simulink model "GSFR_Individual_Vars"  (R2019b)
settings: Solver=VariableStepAuto  StartTime=0  StopTime=20.0  MaxStep=0.01  RelTol=1e-3
model workspace (MAT data in the model file):
  H = [8 1]
values from neighbouring files (symbols this model uses):
  c = (((2*H*R)+(((D*R)+(K*Fh))*Tr))/(2*(D*R+K)))*wn    [Monte_Carlo_Half_Injection.m]    (also in Range_H_Half_Injection.m; Range_H_Ideal_Injection.m)
  D = 1.0    (= 1)    [Monte_Carlo_Half_Injection.m]    (also in Range_H_Half_Injection.m; Range_H_Ideal_Injection.m)
  Fh = 0.034*randn()+0.25    [Monte_Carlo_Half_Injection.m]    (also in Range_H_Half_Injection.m = 0.2; Range_H_Ideal_Injection.m = 0.4)
  K = 0.95    [Monte_Carlo_Half_Injection.m]    (also in Range_H_Half_Injection.m = 0.8; Range_H_Ideal_Injection.m = 1)
  Pd = -0.1    [Monte_Carlo_Half_Injection.m]    (also in Range_H_Half_Injection.m; Range_H_Ideal_Injection.m)
  R = (0.05/3)*randn()+0.075    [Monte_Carlo_Half_Injection.m]    (also in Range_H_Half_Injection.m = 0.075; Range_H_Ideal_Injection.m = 0.04)
  Tr = 0.67*randn()+9    [Monte_Carlo_Half_Injection.m]    (also in Range_H_Half_Injection.m = 8; Range_H_Ideal_Injection.m = 8)
  wn = sqrt((D*R+K)/(2*H*R*Tr))    [Monte_Carlo_Half_Injection.m]    (also in Range_H_Half_Injection.m; Range_H_Ideal_Injection.m)
settings Model: EnablePacing=on  PacingRate=1000  ParameterArgumentNames=H  OrderedModelArguments=off  Creator=ruiva  LastModifiedBy=ruiva

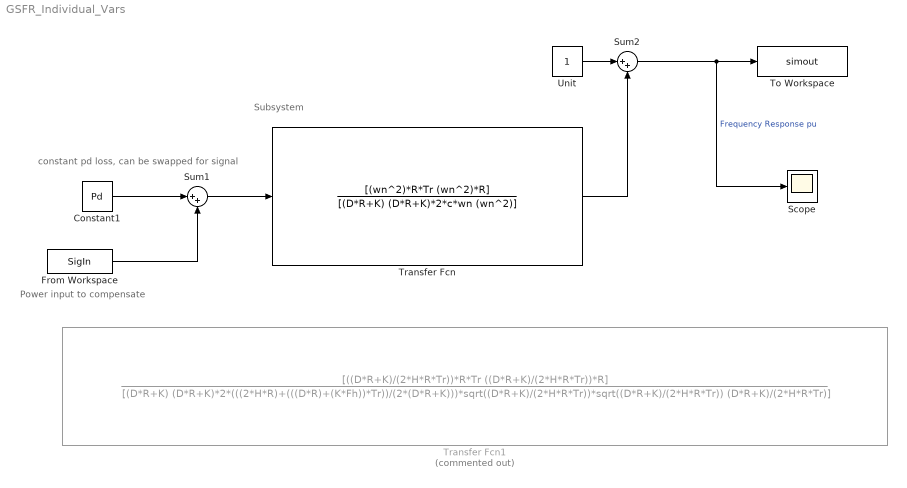
== system GSFR_Individual_Vars ==
  note: Subsystem
  note: Power input to compensate
  note: constant pd loss, can be swapped for signal
  Constant1 : Constant  Value=Pd
  From Workspace : FromWorkspace  VariableName=SigIn  SampleTime=0
  Scope : Scope
  Sum1 : Sum  Inputs=|++
  Sum2 : Sum  Inputs=|++
  To Workspace : ToWorkspace  VariableName=simout  SaveFormat=Timeseries  SampleTime=-1
  Transfer Fcn : TransferFcn  Numerator=[(wn^2)*R*Tr (wn^2)*R]  Denominator=[(D*R+K) (D*R+K)*2*c*wn (wn^2)]
  Transfer Fcn1 : TransferFcn  Commented=on  Numerator=[((D*R+K)/(2*H*R*Tr))*R*Tr ((D*R+K)/(2*H*R*Tr))*R]  Denominator=[(D*R+K) (D*R+K)*2*(((2*H*R)+(((D*R)+(K*Fh))*Tr))/(2*(D*R+K)))*sqrt((D*R+K)/(2*H*R*Tr))*sqrt((D*R+K)/(2*H*R*Tr)) (D*R+K)/(2*H*R*Tr)]
  Unit : Constant
  wires:
  Unit/1 -> Sum2/1
  Sum2/1 -> Scope/1, To Workspace/1  "Frequency Response pu"
  From Workspace/1 -> Sum1/2
  Constant1/1 -> Sum1/1
  Sum1/1 -> Transfer Fcn/1
  Transfer Fcn/1 -> Sum2/2
